simulink model "main"  (R2022a)
settings: Solver=FixedStepDiscrete  StartTime=0.0  StopTime=Inf  FixedStep=(50e-6)-(sim_en*4.995e-5)  RelTol=1e-3  EnableMultiTasking=on
model workspace (MAT data in the model file):
  Param : Simulink.Parameter (value not decoded)
  ac_ok : Simulink.Signal (value not decoded)
  ac_ok_120 : Simulink.Signal (value not decoded)
  bulk_voltage : Simulink.Signal (value not decoded)
  burstduty_integ_max : Simulink.Signal (value not decoded)
  burstduty_integ_min : Simulink.Signal (value not decoded)
  burstduty_ki : Simulink.Signal (value not decoded)
  burstduty_kp : Simulink.Signal (value not decoded)
  calib_ok : Simulink.Signal (value not decoded)
  can_addr1 : Simulink.Signal (value not decoded)
  can_addr2 : Simulink.Signal (value not decoded)
  can_addr3 : Simulink.Signal (value not decoded)
  can_addr4 : Simulink.Signal (value not decoded)
  can_data_rx : Simulink.Signal (value not decoded)
  can_data_tx : Simulink.Signal (value not decoded)
  can_timeout_120 : Simulink.Signal (value not decoded)
  chksum_scircv : Simulink.Signal (value not decoded)
  clllc_en_120 : Simulink.Signal (value not decoded)
  clllc_fault_120 : Simulink.Signal (value not decoded)
  clllc_ok_120 : Simulink.Signal (value not decoded)
  cmpss1h : Simulink.Signal (value not decoded)
  cmpss1l : Simulink.Signal (value not decoded)
  cmpss2h : Simulink.Signal (value not decoded)
  cmpss2l : Simulink.Signal (value not decoded)
  cmpss3h : Simulink.Signal (value not decoded)
  cmpss3l : Simulink.Signal (value not decoded)
  cmpss4h : Simulink.Signal (value not decoded)
  cmpss4l : Simulink.Signal (value not decoded)
  cmpss5h : Simulink.Signal (value not decoded)
  cmpss5l : Simulink.Signal (value not decoded)
  cmpss6h : Simulink.Signal (value not decoded)
  cmpss6l : Simulink.Signal (value not decoded)
  cmpss7h : Simulink.Signal (value not decoded)
  cmpss7l : Simulink.Signal (value not decoded)
  cmpss8h : Simulink.Signal (value not decoded)
  cmpss8l : Simulink.Signal (value not decoded)
  cnt_idle : Simulink.Signal (value not decoded)
  cnt_orps : Simulink.Signal (value not decoded)
  cnt_scircv : Simulink.Signal (value not decoded)
  cnt_scixmt : Simulink.Signal (value not decoded)
  cnt_scixmt_func : Simulink.Signal (value not decoded)
  cnt_temp_mux : Simulink.Signal (value not decoded)
  cnt_vdroop : Simulink.Signal (value not decoded)
  config_ok : Simulink.Signal (value not decoded)
  control_en : Simulink.Signal (value not decoded)
  cp_ready_120 : Simulink.Signal (value not decoded)
  d2d_en : Simulink.Signal (value not decoded)
  dchg_off : Simulink.Signal (value not decoded)
  debug_dacb : Simulink.Signal (value not decoded)
  debug_dacc : Simulink.Signal (value not decoded)
  debug_msg1 : Simulink.Signal (value not decoded)
  debug_msg2 : Simulink.Signal (value not decoded)
  debug_msg3 : Simulink.Signal (value not decoded)
  debug_msg4 : Simulink.Signal (value not decoded)
  debug_msg5 : Simulink.Signal (value not decoded)
  debug_msg6 : Simulink.Signal (value not decoded)
  dir_v2g : Simulink.Signal (value not decoded)
  eoss_llc1 : Simulink.Signal (value not decoded)
  eoss_llc2 : Simulink.Signal (value not decoded)
  eoss_orps : Simulink.Signal (value not decoded)
  fault_ocp : Simulink.Signal (value not decoded)
  fault_otp : Simulink.Signal (value not decoded)
  fault_ovp : Simulink.Signal (value not decoded)
  fut_en : Simulink.Signal (value not decoded)
  fwd_en_120 : Simulink.Signal (value not decoded)
  gain_llc1_sec_idc : Simulink.Signal (value not decoded)
  gain_llc1_temp_sr : Simulink.Signal (value not decoded)
  gain_llc2_sec_idc : Simulink.Signal (value not decoded)
  gain_vbat : Simulink.Signal (value not decoded)
  gain_vbulk : Simulink.Signal (value not decoded)
  gain_vout : Simulink.Signal (value not decoded)
  input_current_phasea : Simulink.Signal (value not decoded)
  input_current_phaseb : Simulink.Signal (value not decoded)
  input_current_phasec : Simulink.Signal (value not decoded)
  input_freq : Simulink.Signal (value not decoded)
  input_power : Simulink.Signal (value not decoded)
  input_voltage_phasea : Simulink.Signal (value not decoded)
  input_voltage_phaseb : Simulink.Signal (value not decoded)
  input_voltage_phasec : Simulink.Signal (value not decoded)
  ishare_arbiter : Simulink.Signal (value not decoded)
  ishare_thresh : Simulink.Signal (value not decoded)
  led_g : Simulink.Signal (value not decoded)
  led_r : Simulink.Signal (value not decoded)
  led_y : Simulink.Signal (value not decoded)
  llc1_burst_integ : Simulink.Signal (value not decoded)
  llc1_burstduty_buffer : Simulink.Signal (value not decoded)
  llc1_pfm_error : Simulink.Signal (value not decoded)
  llc1_pfm_integ : Simulink.Signal (value not decoded)
  llc1_pfm_prop : Simulink.Signal (value not decoded)
  llc1_pri_idc : Simulink.Signal (value not decoded)
  llc1_ps_buffer : Simulink.Signal (value not decoded)
  llc1_pspwm_error : Simulink.Signal (value not decoded)
  llc1_pspwm_integ : Simulink.Signal (value not decoded)
  llc1_pspwm_prop : Simulink.Signal (value not decoded)
  llc1_sec_idc : Simulink.Signal (value not decoded)
  llc1_temp_sr : Simulink.Signal (value not decoded)
  llc1_ts_tbctr_buffer : Simulink.Signal (value not decoded)
  llc2_burst_integ : Simulink.Signal (value not decoded)
  llc2_burstduty_buffer : Simulink.Signal (value not decoded)
  llc2_en : Simulink.Signal (value not decoded)
  llc2_en_buffer : Simulink.Signal (value not decoded)
  llc2_pfm_error : Simulink.Signal (value not decoded)
  llc2_pfm_integ : Simulink.Signal (value not decoded)
  llc2_pfm_prop : Simulink.Signal (value not decoded)
  llc2_pri_idc : Simulink.Signal (value not decoded)
  llc2_ps_buffer : Simulink.Signal (value not decoded)
  llc2_pspwm_error : Simulink.Signal (value not decoded)
  llc2_pspwm_integ : Simulink.Signal (value not decoded)
  llc2_pspwm_prop : Simulink.Signal (value not decoded)
  llc2_sec_idc : Simulink.Signal (value not decoded)
  llc2_temp_sr : Simulink.Signal (value not decoded)
  llc2_ts_tbctr_buffer : Simulink.Signal (value not decoded)
  loop_adcint : Simulink.Signal (value not decoded)
  loop_control : Simulink.Signal (value not decoded)
  loop_idle : Simulink.Signal (value not decoded)
  mid_bulk_voltage : Simulink.Signal (value not decoded)
  mode_120 : Simulink.Signal (value not decoded)
  mode_cc_cv : Simulink.Signal (value not decoded)
  myParam : mpt.Parameter (value not decoded)
  obc_ok_120 : Simulink.Signal (value not decoded)
  offset_llc1_sec_idc : Simulink.Signal (value not decoded)
  offset_llc1_temp_sr : Simulink.Signal (value not decoded)
  offset_llc2_sec_idc : Simulink.Signal (value not decoded)
  offset_vbat : Simulink.Signal (value not decoded)
  offset_vbulk : Simulink.Signal (value not decoded)
  offset_vout : Simulink.Signal (value not decoded)
  openloop_en : Simulink.Signal (value not decoded)
  openloop_fault_en : Simulink.Signal (value not decoded)
  ot_fault_120 : Simulink.Signal (value not decoded)
  pfc_en : Simulink.Signal (value not decoded)
  pfc_en_120 : Simulink.Signal (value not decoded)
  pfc_fw_revision : Simulink.Signal (value not decoded)
  pfc_fw_revision_bootloader : Simulink.Signal (value not decoded)
  pfc_fw_revision_debug : Simulink.Signal (value not decoded)
  pfc_ok : Simulink.Signal (value not decoded)
  pfc_ok_120 : Simulink.Signal (value not decoded)
  pfm_a0 : Simulink.Signal (value not decoded)
  pfm_a1 : Simulink.Signal (value not decoded)
  pfm_integ_max : Simulink.Signal (value not decoded)
  pfm_integ_min : Simulink.Signal (value not decoded)
  pfm_ki : Simulink.Signal (value not decoded)
  pfm_kp : Simulink.Signal (value not decoded)
  pri_fut_en : Simulink.Signal (value not decoded)
  pri_fut_en_buffer : Simulink.Signal (value not decoded)
  pri_halfbridge_en : Simulink.Signal (value not decoded)
  pri_halfbridge_en_buffer : Simulink.Signal (value not decoded)
  pspwm_integ_max : Simulink.Signal (value not decoded)
  pspwm_integ_min : Simulink.Signal (value not decoded)
  pspwm_ki : Simulink.Signal (value not decoded)
  pspwm_kp : Simulink.Signal (value not decoded)
  ref_idclink_max : Simulink.Signal (value not decoded)
  ref_iout : Simulink.Signal (value not decoded)
  ref_iout_calib : Simulink.Signal (value not decoded)
  ref_iout_llc1 : Simulink.Signal (value not decoded)
  ref_iout_llc1_calib : Simulink.Signal (value not decoded)
  ref_iout_llc2 : Simulink.Signal (value not decoded)
  ref_iout_llc2_calib : Simulink.Signal (value not decoded)
  ref_pout : Simulink.Signal (value not decoded)
  ref_ss_llc1 : Simulink.Signal (value not decoded)
  ref_ss_llc2 : Simulink.Signal (value not decoded)
  ref_ss_orps : Simulink.Signal (value not decoded)
  ref_vbat : Simulink.Signal (value not decoded)
  ref_vbat_calib : Simulink.Signal (value not decoded)
  ref_vbulk : Simulink.Signal (value not decoded)
  ref_vbulk_calib : Simulink.Signal (value not decoded)
  ref_vbulk_llc1_calib : Simulink.Signal (value not decoded)
  ref_vbulk_llc2_calib : Simulink.Signal (value not decoded)
  ref_vout : Simulink.Signal (value not decoded)
  ref_vout_calib : Simulink.Signal (value not decoded)
  relay_en : Simulink.Signal (value not decoded)
  reset_flag : Simulink.Signal (value not decoded)
  rev_en_120 : Simulink.Signal (value not decoded)
  runtime_control : Simulink.Signal (value not decoded)
  runtime_idle : Simulink.Signal (value not decoded)
  scircv_buffer : Simulink.Signal (value not decoded)
  scircv_buffer_tmp : Simulink.Signal (value not decoded)
  scircv_buffer_tmp_idx0 : Simulink.Signal (value not decoded)
  scircv_chksum : Simulink.Signal (value not decoded)
  scircv_chksum_ok : Simulink.Signal (value not decoded)
  scircv_parse_ok : Simulink.Signal (value not decoded)
  scixmt_buffer : Simulink.Signal (value not decoded)
  scixmt_chksum : Simulink.Signal (value not decoded)
  scixmt_func : Simulink.Signal (value not decoded)
  scixmt_word0_lsb : Simulink.Signal (value not decoded)
  scixmt_word0_msb : Simulink.Signal (value not decoded)
  scixmt_word1_lsb : Simulink.Signal (value not decoded)
  scixmt_word1_msb : Simulink.Signal (value not decoded)
  scixmt_word2_lsb : Simulink.Signal (value not decoded)
  scixmt_word2_msb : Simulink.Signal (value not decoded)
  scixmt_wr : Simulink.Signal (value not decoded)
  ss_step : Simulink.Signal (value not decoded)
  state_calib : Simulink.Signal (value not decoded)
  state_control : Simulink.Signal (value not decoded)
  state_hkeep : Simulink.Signal (value not decoded)
  status_cmpss : Simulink.Signal (value not decoded)
  status_control : Simulink.Signal (value not decoded)
  status_digin : Simulink.Signal (value not decoded)
  status_digout : Simulink.Signal (value not decoded)
  status_fault : Simulink.Signal (value not decoded)
  status_input : Simulink.Signal (value not decoded)
  status_pfc : Simulink.Signal (value not decoded)
  temp_inlet : Simulink.Signal (value not decoded)
  temp_llc1_fet_hs : Simulink.Signal (value not decoded)
  temp_llc2_fet_hs : Simulink.Signal (value not decoded)
  temp_mux : Simulink.Signal (value not decoded)
  temp_mux_s0 : Simulink.Signal (value not decoded)
  temp_mux_s1 : Simulink.Signal (value not decoded)
  temp_mux_s2 : Simulink.Signal (value not decoded)
  temp_outlet : Simulink.Signal (value not decoded)
  temp_pfc_fet_hsa : Simulink.Signal (value not decoded)
  temp_pfc_fet_hsb : Simulink.Signal (value not decoded)
  temp_pfc_fet_hsc : Simulink.Signal (value not decoded)
  temp_pfc_fet_lsa : Simulink.Signal (value not decoded)
  temp_pfc_fet_lsb : Simulink.Signal (value not decoded)
  temp_pfc_fet_lsc : Simulink.Signal (value not decoded)
  test_mode : Simulink.Signal (value not decoded)
  tfcv_cc : Simulink.Signal (value not decoded)
  tfcv_cc_llc2 : Simulink.Signal (value not decoded)
  tfcv_cv : Simulink.Signal (value not decoded)
  tfcv_sr_en : Simulink.Signal (value not decoded)
  tfv_assert_llc1_pri_idc : Simulink.Signal (value not decoded)
  tfv_assert_llc1_sec_idc : Simulink.Signal (value not decoded)
  tfv_assert_llc1_temp_sr : Simulink.Signal (value not decoded)
  tfv_assert_llc2_pri_idc : Simulink.Signal (value not decoded)
  tfv_assert_llc2_sec_idc : Simulink.Signal (value not decoded)
  tfv_assert_llc2_temp_sr : Simulink.Signal (value not decoded)
  tfv_assert_temp_outlet : Simulink.Signal (value not decoded)
  tfv_assert_vaux_uv : Simulink.Signal (value not decoded)
  tfv_assert_vbat : Simulink.Signal (value not decoded)
  tfv_assert_vbulk : Simulink.Signal (value not decoded)
  tfv_assert_vout : Simulink.Signal (value not decoded)
  tfv_cnt_tz : Simulink.Signal (value not decoded)
  tfv_deassert_llc1_pri_idc : Simulink.Signal (value not decoded)
  tfv_deassert_llc1_sec_idc : Simulink.Signal (value not decoded)
  tfv_deassert_llc1_temp_sr : Simulink.Signal (value not decoded)
  tfv_deassert_llc2_pri_idc : Simulink.Signal (value not decoded)
  tfv_deassert_llc2_sec_idc : Simulink.Signal (value not decoded)
  tfv_deassert_llc2_temp_sr : Simulink.Signal (value not decoded)
  tfv_deassert_temp_outlet : Simulink.Signal (value not decoded)
  tfv_deassert_vaux_uv : Simulink.Signal (value not decoded)
  tfv_deassert_vbat : Simulink.Signal (value not decoded)
  tfv_deassert_vbulk : Simulink.Signal (value not decoded)
  tfv_deassert_vout : Simulink.Signal (value not decoded)
  tfv_llc1_pri_idc : Simulink.Signal (value not decoded)
  tfv_llc1_sec_idc : Simulink.Signal (value not decoded)
  tfv_llc1_temp_sr : Simulink.Signal (value not decoded)
  tfv_llc2_pri_idc : Simulink.Signal (value not decoded)
  tfv_llc2_sec_idc : Simulink.Signal (value not decoded)
  tfv_llc2_temp_sr : Simulink.Signal (value not decoded)
  tfv_temp_outlet : Simulink.Signal (value not decoded)
  tfv_vaux_uv : Simulink.Signal (value not decoded)
  tfv_vbat : Simulink.Signal (value not decoded)
  tfv_vbulk : Simulink.Signal (value not decoded)
  tfv_vout : Simulink.Signal (value not decoded)
  timer_1ms : Simulink.Signal (value not decoded)
  tz : Simulink.Signal (value not decoded)
  valve_en : Simulink.Signal (value not decoded)
  vaux : Simulink.Signal (value not decoded)
  vbat : Simulink.Signal (value not decoded)
  vbulk : Simulink.Signal (value not decoded)
  vout : Simulink.Signal (value not decoded)
undefined symbols (not defined in the file or in its folder): CAN_O_INT, CANA_BASE, Down, GPTRIP1SEL, GPTRIP2SEL, TZ1, TZ2, Up
libraries: hdlsllib x159, simulink x100, c2837xDlib x24, c2807xlib x16, c280xlib x13, c2802xlib x12, canmsglib x8, idelinklib_common x2, c2000lib x1, c281xlib x1
(part 7 of 15)

== system main/Task_Manager/idle/idle_task/uartx/parse ==
  function : TriggerPort  TriggerType=function-call  VariantControl=Variant
  System Outputs3 : Subsystem  mask(System Outputs){ShowInLibBrowser=0}
      mask prompts: ShowInLibBrowser "Simulink:masks:CustCodeMaskParam1_MP"
      settings: CopyFcn=cccopyfcn(gcb)  OpenFcn=ccopenfcn('System Outputs Function')
      mask Help: eval('feval(''rtwprivate'',''rtwhelpview'',''rtw_sys_outputs_block'')');
      mask Display: disp('System\nOutputs');

== system main/Task_Manager/idle/idle_task/uartx/uart_xmt ==
  function : TriggerPort  TriggerType=function-call  VariantControl=Variant

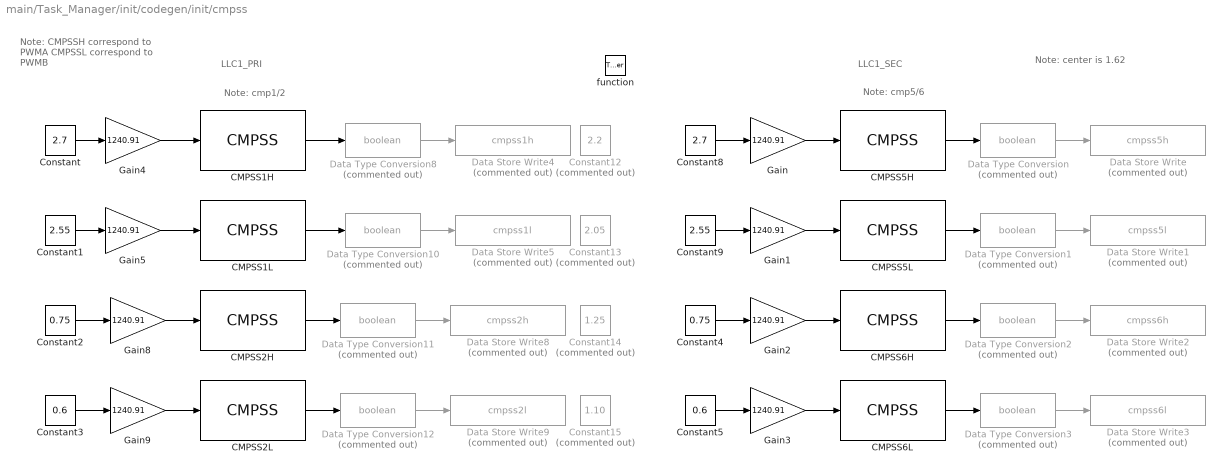
== system main/Task_Manager/init/codegen/init/cmpss ==
  note: Note:
      | center is 1.62
  note: Note:
      | CMPSSH correspond to PWMA
      | CMPSSL correspond to PWMB
  note: LLC1_PRI
  note: LLC1_SEC
  note: Note: cmp1/2
  note: Note: cmp5/6
  function : TriggerPort  TriggerType=function-call  VariantControl=Variant
  CMPSS1H : c2837xDlib/CMPSS  Module=CMPSS1_COMPH  NegativeInput=Internal DAC  DacValueSourceSel=DAC module  DacValueVia=Input port  DACHValue=2234  DACLValue=0  RampMaxRefVal=0  RampDecVal=0  RampDelayVal=0  EnableLatchOut=off  EnableLatchClear=off  SampleTime=-1
      settings: SourceProductBaseCode=TIC2000
  CMPSS1L : c2837xDlib/CMPSS  Module=CMPSS1_COMPL  NegativeInput=Internal DAC  DacValueSourceSel=DAC module  DacValueVia=Input port  DACHValue=2234  DACLValue=0  RampMaxRefVal=0  RampDecVal=0  RampDelayVal=0  EnableLatchOut=off  EnableLatchClear=off  SampleTime=-1
      settings: SourceProductBaseCode=TIC2000
  CMPSS2H : c2837xDlib/CMPSS  Module=CMPSS2_COMPH  NegativeInput=Internal DAC  DacValueSourceSel=DAC module  DacValueVia=Input port  DACHValue=2234  DACLValue=0  RampMaxRefVal=0  RampDecVal=0  RampDelayVal=0  EnableLatchOut=off  EnableLatchClear=off  SampleTime=-1
      settings: SourceProductBaseCode=TIC2000
  CMPSS2L : c2837xDlib/CMPSS  Module=CMPSS2_COMPL  NegativeInput=Internal DAC  DacValueSourceSel=DAC module  DacValueVia=Input port  DACHValue=2234  DACLValue=0  RampMaxRefVal=0  RampDecVal=0  RampDelayVal=0  EnableLatchOut=off  EnableLatchClear=off  SampleTime=-1
      settings: SourceProductBaseCode=TIC2000
  CMPSS5H : c2837xDlib/CMPSS  Module=CMPSS5_COMPH  NegativeInput=Internal DAC  DacValueSourceSel=DAC module  DacValueVia=Input port  DACHValue=2234  DACLValue=0  RampMaxRefVal=0  RampDecVal=0  RampDelayVal=0  EnableLatchOut=off  EnableLatchClear=off  SampleTime=-1
      settings: SourceProductBaseCode=TIC2000
  CMPSS5L : c2837xDlib/CMPSS  Module=CMPSS5_COMPL  NegativeInput=Internal DAC  DacValueSourceSel=DAC module  DacValueVia=Input port  DACHValue=2234  DACLValue=0  RampMaxRefVal=0  RampDecVal=0  RampDelayVal=0  EnableLatchOut=off  EnableLatchClear=off  SampleTime=-1
      settings: SourceProductBaseCode=TIC2000
  CMPSS6H : c2837xDlib/CMPSS  Module=CMPSS6_COMPH  NegativeInput=Internal DAC  DacValueSourceSel=DAC module  DacValueVia=Input port  DACHValue=2234  DACLValue=0  RampMaxRefVal=0  RampDecVal=0  RampDelayVal=0  EnableLatchOut=off  EnableLatchClear=off  SampleTime=-1
      settings: SourceProductBaseCode=TIC2000
  CMPSS6L : c2837xDlib/CMPSS  Module=CMPSS6_COMPL  NegativeInput=Internal DAC  DacValueSourceSel=DAC module  DacValueVia=Input port  DACHValue=2234  DACLValue=0  RampMaxRefVal=0  RampDecVal=0  RampDelayVal=0  EnableLatchOut=off  EnableLatchClear=off  SampleTime=-1
      settings: SourceProductBaseCode=TIC2000
  Constant : Constant  Value=2.7
  Constant1 : Constant  Value=2.55
  Constant12 : Constant  Commented=on  Value=2.2
  Constant13 : Constant  Commented=on  Value=2.05
  Constant14 : Constant  Commented=on  Value=1.25
  Constant15 : Constant  Commented=on  Value=1.10
  Constant2 : Constant  Value=0.75
  Constant3 : Constant  Value=0.6
  Constant4 : Constant  Value=0.75
  Constant5 : Constant  Value=0.6
  Constant8 : Constant  Value=2.7
  Constant9 : Constant  Value=2.55
  Data Store Write : DataStoreWrite  Commented=on  DataStoreName=cmpss5h  IndexOptions=Index vector (dialog)  Indices=1  OutputSizes=1
  Data Store Write1 : DataStoreWrite  Commented=on  DataStoreName=cmpss5l  IndexOptions=Index vector (dialog)  Indices=1  OutputSizes=1
  Data Store Write2 : DataStoreWrite  Commented=on  DataStoreName=cmpss6h  IndexOptions=Index vector (dialog)  Indices=1  OutputSizes=1
  Data Store Write3 : DataStoreWrite  Commented=on  DataStoreName=cmpss6l  IndexOptions=Index vector (dialog)  Indices=1  OutputSizes=1
  Data Store Write4 : DataStoreWrite  Commented=on  DataStoreName=cmpss1h  IndexOptions=Index vector (dialog)  Indices=1  OutputSizes=1
  Data Store Write5 : DataStoreWrite  Commented=on  DataStoreName=cmpss1l  IndexOptions=Index vector (dialog)  Indices=1  OutputSizes=1
  Data Store Write8 : DataStoreWrite  Commented=on  DataStoreName=cmpss2h  IndexOptions=Index vector (dialog)  Indices=1  OutputSizes=1
  Data Store Write9 : DataStoreWrite  Commented=on  DataStoreName=cmpss2l  IndexOptions=Index vector (dialog)  Indices=1  OutputSizes=1
  Data Type Conversion{,1..3,8,10..12} (8 alike) : DataTypeConversion  Commented=on  OutDataTypeStr=boolean  SaturateOnIntegerOverflow=off  RndMeth=Floor
  Gain{,1..5,8..9} (8 alike) : Gain  Gain=1240.91
  wires:
  Constant/1 -> Gain4/1
  Constant1/1 -> Gain5/1
  Gain/1 -> CMPSS5H/1
  Gain1/1 -> CMPSS5L/1
  Gain2/1 -> CMPSS6H/1
  Gain3/1 -> CMPSS6L/1
  CMPSS5H/1 -> Data Type Conversion/1
  CMPSS5L/1 -> Data Type Conversion1/1
  CMPSS6H/1 -> Data Type Conversion2/1
  CMPSS6L/1 -> Data Type Conversion3/1
  CMPSS1H/1 -> Data Type Conversion8/1
  CMPSS1L/1 -> Data Type Conversion10/1
  Gain4/1 -> CMPSS1H/1
  Gain5/1 -> CMPSS1L/1
  CMPSS2L/1 -> Data Type Conversion12/1
  CMPSS2H/1 -> Data Type Conversion11/1
  Gain9/1 -> CMPSS2L/1
  Gain8/1 -> CMPSS2H/1
  Constant3/1 -> Gain9/1
  Constant2/1 -> Gain8/1
  Data Type Conversion/1 -> Data Store Write/1
  Data Type Conversion1/1 -> Data Store Write1/1
  Data Type Conversion3/1 -> Data Store Write3/1
  Data Type Conversion2/1 -> Data Store Write2/1
  Data Type Conversion8/1 -> Data Store Write4/1
  Data Type Conversion10/1 -> Data Store Write5/1
  Data Type Conversion11/1 -> Data Store Write8/1
  Data Type Conversion12/1 -> Data Store Write9/1
  Constant4/1 -> Gain2/1
  Constant5/1 -> Gain3/1
  Constant9/1 -> Gain1/1
  Constant8/1 -> Gain/1

== system main/Task_Manager/init/codegen/init/orps&relay ==
  note: Note:
      | Period: 100kHz
      |
      | Timer Period: 1000
      |
      | ePWM9 GPIO16
  function : TriggerPort  TriggerType=function-call  VariantControl=Variant
  ORPS : c2802xlib/ePWM  PwmType=C2000_Type4  useModule=ePWM9  ePWMxLINKTBPRD=Not Linked  periodUnits=Clock cycles  timerSource=Specify via dialog  timerPeriod_clk=1000  timerPeriod_sec=0.0001  tbshadow=Counter equals to zero  countingMode=Up-Down  phaseActiveEnable=Disable  phaseDirection=Count down after sync  phaseActive=0  synchronizationEnable=off  dcaevt1Sync=off  dcbevt1Sync=off  synchronizationOption=Pass through (EPWMxSYNCI or SWFSYNC)  perSynchronizationOption=Counter equals to period (CTR=PRD)  clockPrescale=1  HSclockPrescale=1  enswap=off  ePWMxAStatus=on  ePWMxAactionLogic1=Set  ePWMxAactionLogic2=Do nothing  ePWMxAactionLogic3=Do nothing  ePWMxAactionLogic4=Do nothing  ePWMxAactionLogic5=Clear  ePWMxAactionLogic6=Do nothing  ePWMxACSFenable=off  ePWMxACSFvalue=Forcing disable  ePWMxASFreload=Zero  ePWMxBStatus=on  ePWMxBactionLogic1=Do nothing  ePWMxBactionLogic2=Set  ePWMxBactionLogic3=Do nothing  ePWMxBactionLogic4=Clear  ePWMxBactionLogic5=Do nothing  ePWMxBactionLogic6=Do nothing  ePWMxBCSFenable=off  ePWMxBCSFvalue=Forcing disable  ePWMxBSFreload=Zero  ePWNxBOutWay=off  ePWMxLINKCMPA=Not Linked  CMPAUnits=Clock cycles  CMPASource=Specify via dialog  CMPAValue_per=50  CMPAValue_clk=5  enCMPAshadow=Counter equals to zero (CTR=Zero)  ePWMxLINKCMPB=Not Linked  CMPBUnits=Clock cycles  CMPBSource=Specify via dialog  CMPBValue_per=50  CMPBValue_clk=995  enCMPBshadow=Counter equals to zero (CTR=Zero)  ePWMxLINKCMPC=Not Linked  CMPCUnits=Clock cycles  CMPCSource=Specify via dialog  CMPCValue_per=50  CMPCValue_clk=0  enCMPCshadow=Counter equals to zero (CTR=Zero)  ePWMxLINKCMPD=Not Linked  CMPDUnits=Clock cycles  CMPDSource=Specify via dialog  CMPDValue_per=50  CMPDValue_clk=0  enCMPDshadow=Counter equals to zero (CTR=Zero)  enableDBePWMxA=off  enableDBePWMxB=off  enhalfcycle=off  DBpolarity=Active high complementary (AHC)  DBedgeDelay=Positive  DBSource_ePWMxA=ePWMxA  DBSource_ePWMxB=ePWMxA  DBPeriodUnits=Clock cycles  DBperiodSource=Input port  REDperiod=36  FEDperiod=36  REDperiod_sec=0  FEDperiod_sec=0  LoadModeDBRED=Immediate without using shadow  LoadModeDBFED=Immediate without using shadow  adcstartModuleA=off  adcrequestEventA=First event  adcstartEventA=Digital Compare Module A Event 1 start of conversion (DCAEVT1.soc)  adcstartEventA_type2=Counter is incrementing and equals to the compare B register (CTRU=CMPB)  adcstartModuleB=off  adcrequestEventB=First event  adcstartEventB=Counter equals to zero (CTR=Zero)  adcstartEventB_type2=Counter is incrementing and equals to the compare B register (CTRU=CMPB)  intEn=off  intPrd=First event  intSel=Counter equals to zero (CTR=Zero)  intSel_type2=Counter equals to zero (CTR=Zero)  hrpe=off  enHRPWM=off  HRPWM_LoadMode=Counter equals to period (CTR=PRD)  HRPWM_CTLMode=Duty or Period control mode  HRPWM_EDGMode=Both edge  hrpeb=off  enHRPWMB=off  HRPWM_LoadModeB=Counter equals to zero (CTR=ZERO)  HRPWM_CTLModeB=Duty or Period control mode  HRPWM_EDGModeB=Both edge  enHRDBRED=off  enHRDBFED=off  enSFO=on  enautoconv=on  chopperEnable=off  chopperFrequency=1  chopperFirstwidth=1  chopperDuty=12.5%  tripZonesource=Specify via dialog  tzselOSHT1=off  tzselOSHT2=off  tzselOSHT3=off  tzselOSHDCAEV1=off  tzselOSHDCBEV1=off  tzselCBC1=off  tzselCBC2=off  tzselCBC3=off  tzselCBCDCAEV2=off  tzselCBCDCBEV2=off  tzselOSHT4=off  tzselOSHT5=off  tzselOSHT6=off  tzselCBC4=off  tzselCBC5=off  tzselCBC6=off  enTzOstIntr=off  enTzCbcIntr=off  enTzDCAEVT1Intr=off  enTzDCAEVT2Intr=off  enTzDCBEVT1Intr=off  enTzDCBEVT2Intr=off  ePWMxAforced=No action  ePWMxBforced=No action  DCAEVT1forced=High  DCBEVT1forced=Low  DCAEVT2forced=Low  DCBEVT2forced=High  dcah=Trip Zone 1 input (TZ1)  dcal=Trip Zone 2 input (TZ2)  dcbh=Trip Zone 1 input (TZ1)  dcbl=Trip Zone 2 input (TZ2)  dcah_type2=GPTRIP4SEL  dcal_type2=GPTRIP4SEL  dcbh_type2=GPTRIP5SEL  dcbl_type2=GPTRIP5SEL  gendcaevt1=Event disabled  gendcaevt2=Event disabled  gendcbevt1=Event disabled  gendcbevt2=Event disabled  dcaevt1src=DCAEVT1 with sync  dcaevt2src=DCAEVT2 with sync  dcbevt1src=DCBEVT1 with sync  dcbevt2src=DCBEVT2 with sync  pulsesel=Counter equals to zero (CTR=Zero)  blankinv=off  blankoffset=0  blankwidth=0  evsrcsel=Filtered version of DCAEVT1 (DCAEVT1FILT)  encape=off

== system main/Task_Manager/init/codegen/init/outputxbar ==
  note: //Code:
      | GPIO_setPinConfig(GPIO_24_OUTPUTXBAR1);
      | GPIO_setDirectionMode(24, GPIO_DIR_MODE_OUT);
      | GPIO_setPadConfig(24, GPIO_PIN_TYPE_STD);
      | XBAR_setOutputMuxConfig(XBAR_OUTPUT1, XBAR_OUT_MUX00_CMPSS1_CTRIPOUTH);
      | XBAR_enableOutputMux(XBAR_OUTPUT1, XBAR_MUX00);
      |
      | GPIO_setPinConfig(GPIO_25_OUTPUTXBAR2);
      | GPIO_setDirectionMode(25, GPIO_DIR_MODE_OUT);
      | GPIO_setPadConfig(25, GPIO_PIN_TYPE_STD);
      | XBAR_setOutputMuxConfig(XBAR_OUTPUT2, XBAR_OUT_MUX01_CMPSS1_CTRIPOUTL);
      | XBAR_enableOutputMux(XBAR_OUTPUT2, XBAR_MUX01);
      |
      | GPIO_setPinConfig(GPIO_26_OUTPUTXBAR3);
      | GPIO_setDirectionMode(26, GPIO_DIR_MODE_OUT);
      | GPIO_setPadConfig(26, GPIO_PIN_TYPE_STD);
      | XBAR_setOutputMuxConfig(XBAR_OUTPUT3, XBAR_OUT_MUX04_CMPSS3_CTRIPOUTH);
      | XBAR_enableOutputMux(XBAR_OUTPUT3, XBAR_MUX04);
      |
      | GPIO_setPinConfig(GPIO_27_OUTPUTXBAR4);
      | GPIO_setDirectionMode(27, GPIO_DIR_MODE_OUT);
      | GPIO_setPadConfig(27, GPIO_PIN_TYPE_STD);
      | XBAR_setOutputMuxConfig(XBAR_OUTPUT4, XBAR_OUT_MUX05_CMPSS3_CTRIPOUTL);
      | XBAR_enableOutputMux(XBAR_OUTPUT4, XBAR_MUX05);
  note: GPIO_setPinConfig(GPIO_24_OUTPUTXBAR1);
      | GPIO_setDirectionMode(24, GPIO_DIR_MODE_OUT);
      | GPIO_setPadConfig(24, GPIO_PIN_TYPE_STD);
      | XBAR_setOutputMuxConfig(XBAR_OUTPUT1, XBAR_OUT_MUX11_CMPSS6_CTRIPOUTL);
      | XBAR_enableOutputMux(XBAR_OUTPUT1, XBAR_MUX11);
      |
      | GPIO_setPinConfig(GPIO_25_OUTPUTXBAR2);
      | GPIO_setDirectionMode(25, GPIO_DIR_MODE_OUT);
      | GPIO_setPadConfig(25, GPIO_PIN_TYPE_STD);
      | XBAR_setOutputMuxConfig(XBAR_OUTPUT2, XBAR_OUT_MUX10_CMPSS6_CTRIPOUTH);
      | XBAR_enableOutputMux(XBAR_OUTPUT2, XBAR_MUX10);
  note: GPIO_setPinConfig(GPIO_24_OUTPUTXBAR1);
      | GPIO_setDirectionMode(24, GPIO_DIR_MODE_OUT);
      | GPIO_setPadConfig(24, GPIO_PIN_TYPE_STD);
      | XBAR_setOutputMuxConfig(XBAR_OUTPUT1, XBAR_CLB_MUX08_CMPSS5_CTRIPH);
      | XBAR_enableOutputMux(XBAR_OUTPUT1, XBAR_MUX08);
  note: GPIO_setPinConfig(GPIO_24_OUTPUTXBAR1);
      | GPIO_setDirectionMode(24, GPIO_DIR_MODE_OUT);
      | GPIO_setPadConfig(24, GPIO_PIN_TYPE_STD);
      | XBAR_setOutputMuxConfig(XBAR_OUTPUT1, XBAR_CLB_MUX00_CMPSS1_CTRIPH);
      | XBAR_enableOutputMux(XBAR_OUTPUT1, XBAR_MUX00);
  note: GPIO_setPinConfig(GPIO_25_OUTPUTXBAR2);
      | GPIO_setDirectionMode(25, GPIO_DIR_MODE_OUT);
      | GPIO_setPadConfig(25, GPIO_PIN_TYPE_STD);
      | XBAR_setOutputMuxConfig(XBAR_OUTPUT2, XBAR_CLB_MUX00_CMPSS1_CTRIPH);
      | XBAR_enableOutputMux(XBAR_OUTPUT2, XBAR_MUX00);
  note: GPIO_setPinConfig(GPIO_25_OUTPUTXBAR2);
      | GPIO_setDirectionMode(25, GPIO_DIR_MODE_OUT);
      | GPIO_setPadConfig(25, GPIO_PIN_TYPE_STD);
      | XBAR_setOutputMuxConfig(XBAR_OUTPUT2, XBAR_CLB_MUX08_CMPSS5_CTRIPH);
      | XBAR_enableOutputMux(XBAR_OUTPUT2, XBAR_MUX08);
  function : TriggerPort  TriggerType=function-call  VariantControl=Variant
  System Initialize1 : Subsystem  Commented=on  mask(System Initialize){ShowInLibBrowser=0}
      mask prompts: ShowInLibBrowser "Simulink:masks:CustCodeMaskParam1_MP"
      settings: CopyFcn=cccopyfcn(gcb)  OpenFcn=ccopenfcn('System Initialize Function')
      mask Help: eval('feval(''rtwprivate'',''rtwhelpview'',''rtw_sys_initialize_block'')');
      mask Display: disp('System\nInitialize');
  System Initialize2 : Subsystem  Commented=on  mask(System Initialize){ShowInLibBrowser=0}
      mask prompts: ShowInLibBrowser "Simulink:masks:CustCodeMaskParam1_MP"
      settings: CopyFcn=cccopyfcn(gcb)  OpenFcn=ccopenfcn('System Initialize Function')
      mask Help: eval('feval(''rtwprivate'',''rtwhelpview'',''rtw_sys_initialize_block'')');
      mask Display: disp('System\nInitialize');
  System Initialize3 : Subsystem  Commented=on  mask(System Initialize){ShowInLibBrowser=0}
      mask prompts: ShowInLibBrowser "Simulink:masks:CustCodeMaskParam1_MP"
      settings: CopyFcn=cccopyfcn(gcb)  OpenFcn=ccopenfcn('System Initialize Function')
      mask Help: eval('feval(''rtwprivate'',''rtwhelpview'',''rtw_sys_initialize_block'')');
      mask Display: disp('System\nInitialize');
  System Initialize4 : Subsystem  Commented=on  mask(System Initialize){ShowInLibBrowser=0}
      mask prompts: ShowInLibBrowser "Simulink:masks:CustCodeMaskParam1_MP"
      settings: CopyFcn=cccopyfcn(gcb)  OpenFcn=ccopenfcn('System Initialize Function')
      mask Help: eval('feval(''rtwprivate'',''rtwhelpview'',''rtw_sys_initialize_block'')');
      mask Display: disp('System\nInitialize');
  System Initialize5 : Subsystem  Commented=on  mask(System Initialize){ShowInLibBrowser=0}
      mask prompts: ShowInLibBrowser "Simulink:masks:CustCodeMaskParam1_MP"
      settings: CopyFcn=cccopyfcn(gcb)  OpenFcn=ccopenfcn('System Initialize Function')
      mask Help: eval('feval(''rtwprivate'',''rtwhelpview'',''rtw_sys_initialize_block'')');
      mask Display: disp('System\nInitialize');
  System Initialize6 : Subsystem  mask(System Initialize){ShowInLibBrowser=0}
      mask prompts: ShowInLibBrowser "Simulink:masks:CustCodeMaskParam1_MP"
      settings: CopyFcn=cccopyfcn(gcb)  OpenFcn=ccopenfcn('System Initialize Function')
      mask Help: eval('feval(''rtwprivate'',''rtwhelpview'',''rtw_sys_initialize_block'')');
      mask Display: disp('System\nInitialize');

== system main/Task_Manager/init/codegen/init/pwmsync ==
  note: EALLOW;
      | XBAR_setInputPin(XBAR_INPUT5, 4); //EXTSYNC1 from PWM3A
      | XBAR_setInputPin(XBAR_INPUT6, 10); //EXTSYNC2 from PWM6A
      | EDIS;
  note: Note:
      | grouping is:
      |
      | 1/2            7/8
      |
      | 4/5            10/11
  note: EALLOW;
      | SyncSocRegs.SYNCSELECT.bit.EPWM4SYNCIN = 0b110; //Sync to PWM4 group to EXTSYNC2
      | EDIS;
  note: EALLOW;
      | XBAR_setInputPin(XBAR_INPUT5, 4); //EXTSYNC1 from PWM3A
      | SyncSocRegs.SYNCSELECT.bit.EPWM7SYNCIN = 0b101; //Sync PWM7 group to EXTSYNC1
      | EDIS;
  note: Note:
      | grouping is:
      | Use external sync
      |
      | 1/2            7/8
      |
      | epwm9 for orps
  function : TriggerPort  TriggerType=function-call  VariantControl=Variant
  System Initialize : Subsystem  Commented=on  mask(System Initialize){ShowInLibBrowser=0}
      mask prompts: ShowInLibBrowser "Simulink:masks:CustCodeMaskParam1_MP"
      settings: CopyFcn=cccopyfcn(gcb)  OpenFcn=ccopenfcn('System Initialize Function')
      mask Help: eval('feval(''rtwprivate'',''rtwhelpview'',''rtw_sys_initialize_block'')');
      mask Display: disp('System\nInitialize');
  System Initialize1 : Subsystem  Commented=on  mask(System Initialize){ShowInLibBrowser=0}
      mask prompts: ShowInLibBrowser "Simulink:masks:CustCodeMaskParam1_MP"
      settings: CopyFcn=cccopyfcn(gcb)  OpenFcn=ccopenfcn('System Initialize Function')
      mask Help: eval('feval(''rtwprivate'',''rtwhelpview'',''rtw_sys_initialize_block'')');
      mask Display: disp('System\nInitialize');
  System Initialize2 : Subsystem  mask(System Initialize){ShowInLibBrowser=0}
      mask prompts: ShowInLibBrowser "Simulink:masks:CustCodeMaskParam1_MP"
      settings: CopyFcn=cccopyfcn(gcb)  OpenFcn=ccopenfcn('System Initialize Function')
      mask Help: eval('feval(''rtwprivate'',''rtwhelpview'',''rtw_sys_initialize_block'')');
      mask Display: disp('System\nInitialize');

== system main/Task_Manager/init/codegen/init/tztl_clb ==
  note: Note:
      | Initial configuration is for
      | G2V full-bridge
  function : TriggerPort  TriggerType=function-call  VariantControl=Variant
  Function-Call Generator1 : simulink/Ports & Subsystems/Function-Call Generator  sample_time=-1  numberOfIterations=1  DisallowWideOutput=off
  Function-Call Split3 : FunctionCallSplit  NumOutputPorts=2
  clb : Subsystem  TreatAsAtomicUnit=on
      settings: RTWSystemCode=Inline
  tzctl : Subsystem  TreatAsAtomicUnit=on
      settings: RTWSystemCode=Inline
  wires:
  Function-Call Split3/2 -> clb/Trigger
  Function-Call Generator1/1 -> Function-Call Split3/1
  Function-Call Split3/1 -> tzctl/Trigger

== system main/interrupt_adcd/burst_control/burst/enPulse/Forward/System Outputs1 ==

== system main/interrupt_adcd/burst_control/burst/enPulse/Reverse/System Outputs1 ==

== system main/interrupt_canrx/canrx_variant_subsystem/codegen/can_rcv/Switch Case Action Subsystem ==
  Action Port : ActionPort  ActionPortLabel=case [ 10 ]:
  Constant : Constant  OutDataTypeStr=boolean
  Data Store Write : DataStoreWrite  DataStoreName=u8CanDataRx10  IndexOptions=Index vector (dialog)  Indices=1  OutputSizes=1
  Data Store Write1 : DataStoreWrite  DataStoreName=b05_MB10Received  IndexOptions=Index vector (dialog)  Indices=1  OutputSizes=1
  Terminator : Terminator
  eCAN Receive : c280xlib/eCAN Receive  chipFamily=C280x  useModule=eCAN_A  mailboxNo=9  messageID=hex2dec('00000100')  messageType=Standard (11-bit identifier)  enableAcceptanceFiltering=off  messageIDMask=0  sampleTime=-1  dataType=uint8  outputAction=Output last received values  initValue=0  outputMessageID=off  outputMessageLength=off  outputMessageTimeStamp=off  postInterrupt=on  interruptLine=0
      settings: SourceProductBaseCode=TIC2000
  wires:
  eCAN Receive/2 -> Data Store Write/1
  eCAN Receive/1 -> Terminator/1
  Constant/1 -> Data Store Write1/1

== system main/interrupt_canrx/canrx_variant_subsystem/codegen/can_rcv/Switch Case Action Subsystem1 ==
  Action Port : ActionPort  ActionPortLabel=case [ 11 ]:
  Constant2 : Constant  OutDataTypeStr=boolean
  Data Store Write1 : DataStoreWrite  DataStoreName=b06_MB11Received  IndexOptions=Index vector (dialog)  Indices=1  OutputSizes=1
  Data Store Write3 : DataStoreWrite  DataStoreName=u8CanDataRx11  IndexOptions=Index vector (dialog)  Indices=1  OutputSizes=1
  Terminator1 : Terminator
  eCAN Receive1 : c280xlib/eCAN Receive  chipFamily=C280x  useModule=eCAN_A  mailboxNo=10  messageID=hex2dec('00000102')  messageType=Standard (11-bit identifier)  enableAcceptanceFiltering=off  messageIDMask=0  sampleTime=-1  dataType=uint8  outputAction=Output last received values  initValue=0  outputMessageID=off  outputMessageLength=off  outputMessageTimeStamp=off  postInterrupt=on  interruptLine=0
      settings: SourceProductBaseCode=TIC2000
  wires:
  eCAN Receive1/1 -> Terminator1/1
  eCAN Receive1/2 -> Data Store Write3/1
  Constant2/1 -> Data Store Write1/1

== system main/interrupt_canrx/canrx_variant_subsystem/codegen/can_rcv/Switch Case Action Subsystem2 ==
  Action Port : ActionPort  ActionPortLabel=case [ 12 ]:
  Constant2 : Constant  OutDataTypeStr=boolean
  Data Store Write1 : DataStoreWrite  DataStoreName=u8CanDataRx12  IndexOptions=Index vector (dialog)  Indices=1  OutputSizes=1
  Data Store Write2 : DataStoreWrite  DataStoreName=b07_MB12Received  IndexOptions=Index vector (dialog)  Indices=1  OutputSizes=1
  Terminator2 : Terminator
  eCAN Receive2 : c280xlib/eCAN Receive  chipFamily=C280x  useModule=eCAN_A  mailboxNo=11  messageID=hex2dec('0000010A')  messageType=Standard (11-bit identifier)  enableAcceptanceFiltering=off  messageIDMask=0  sampleTime=-1  dataType=uint8  outputAction=Output last received values  initValue=0  outputMessageID=off  outputMessageLength=off  outputMessageTimeStamp=off  postInterrupt=on  interruptLine=0
      settings: SourceProductBaseCode=TIC2000
  wires:
  eCAN Receive2/1 -> Terminator2/1
  eCAN Receive2/2 -> Data Store Write1/1
  Constant2/1 -> Data Store Write2/1

== system main/Control_State_Machine/Control_Loop/control/configSr/configXbarEpwmtrip/codegen/g2v_prifullbridge ==
  Action Port : ActionPort
  Function-Call Generator1 : simulink/Ports & Subsystems/Function-Call Generator  sample_time=-1  numberOfIterations=1  DisallowWideOutput=off
  Function-Call Split3 : FunctionCallSplit  NumOutputPorts=2
  clb : Subsystem  TreatAsAtomicUnit=on
      settings: RTWSystemCode=Inline
  tzctl : Subsystem  TreatAsAtomicUnit=on
      settings: RTWSystemCode=Inline
  wires:
  Function-Call Split3/1 -> tzctl/Trigger
  Function-Call Generator1/1 -> Function-Call Split3/1
  Function-Call Split3/2 -> clb/Trigger

== system main/Control_State_Machine/Control_Loop/control/configSr/configXbarEpwmtrip/codegen/v2g_prifullbridge ==
  Action Port : ActionPort
  Function-Call Generator2 : simulink/Ports & Subsystems/Function-Call Generator  sample_time=-1  numberOfIterations=1  DisallowWideOutput=off
  Function-Call Split1 : FunctionCallSplit  NumOutputPorts=2
  clb : Subsystem  TreatAsAtomicUnit=on
      settings: RTWSystemCode=Inline
  tzctl : Subsystem  TreatAsAtomicUnit=on
      settings: RTWSystemCode=Inline
  wires:
  Function-Call Generator2/1 -> Function-Call Split1/1
  Function-Call Split1/1 -> tzctl/Trigger
  Function-Call Split1/2 -> clb/Trigger

== system main/Control_State_Machine/Control_Loop/control/configSr/configXbarEpwmtrip/sim/g2v_prifullbridge ==
  Action Port : ActionPort
  Constant{,1..3} (4 alike) : Constant  Value=0  OutDataTypeStr=uint16
  Constant{4,9..11} (4 alike) : Constant  OutDataTypeStr=uint16
  Data Store Write1 : DataStoreWrite  DataStoreName=xbar_epwmtrip_llc1_pri_qb_en  IndexOptions=Index vector (dialog)  Indices=1  OutputSizes=1
  Data Store Write10 : DataStoreWrite  DataStoreName=xbar_epwmtrip_llc1_sec_qd_en  IndexOptions=Index vector (dialog)  Indices=1  OutputSizes=1
  Data Store Write2 : DataStoreWrite  DataStoreName=xbar_epwmtrip_llc1_pri_qc_en  IndexOptions=Index vector (dialog)  Indices=1  OutputSizes=1
  Data Store Write3 : DataStoreWrite  DataStoreName=xbar_epwmtrip_llc1_pri_qd_en  IndexOptions=Index vector (dialog)  Indices=1  OutputSizes=1
  Data Store Write4 : DataStoreWrite  DataStoreName=xbar_epwmtrip_llc1_sec_qa_en  IndexOptions=Index vector (dialog)  Indices=1  OutputSizes=1
  Data Store Write6 : DataStoreWrite  DataStoreName=xbar_epwmtrip_llc1_pri_qa_en  IndexOptions=Index vector (dialog)  Indices=1  OutputSizes=1
  Data Store Write8 : DataStoreWrite  DataStoreName=xbar_epwmtrip_llc1_sec_qb_en  IndexOptions=Index vector (dialog)  Indices=1  OutputSizes=1
  Data Store Write9 : DataStoreWrite  DataStoreName=xbar_epwmtrip_llc1_sec_qc_en  IndexOptions=Index vector (dialog)  Indices=1  OutputSizes=1
  wires:
  Constant3/1 -> Data Store Write3/1
  Constant2/1 -> Data Store Write2/1
  Constant1/1 -> Data Store Write1/1
  Constant/1 -> Data Store Write6/1
  Constant4/1 -> Data Store Write4/1
  Constant9/1 -> Data Store Write8/1
  Constant10/1 -> Data Store Write9/1
  Constant11/1 -> Data Store Write10/1

== system main/Control_State_Machine/Control_Loop/control/configSr/configXbarEpwmtrip/sim/v2g_prifullbridge ==
  Action Port : ActionPort
  Constant{,1..3} (4 alike) : Constant  Value=0  OutDataTypeStr=uint16
  Constant{4,9..11} (4 alike) : Constant  OutDataTypeStr=uint16
  Data Store Write1 : DataStoreWrite  DataStoreName=xbar_epwmtrip_llc1_pri_qb_en  IndexOptions=Index vector (dialog)  Indices=1  OutputSizes=1
  Data Store Write10 : DataStoreWrite  DataStoreName=xbar_epwmtrip_llc1_sec_qd_en  IndexOptions=Index vector (dialog)  Indices=1  OutputSizes=1
  Data Store Write2 : DataStoreWrite  DataStoreName=xbar_epwmtrip_llc1_pri_qc_en  IndexOptions=Index vector (dialog)  Indices=1  OutputSizes=1
  Data Store Write3 : DataStoreWrite  DataStoreName=xbar_epwmtrip_llc1_pri_qd_en  IndexOptions=Index vector (dialog)  Indices=1  OutputSizes=1
  Data Store Write4 : DataStoreWrite  DataStoreName=xbar_epwmtrip_llc1_sec_qa_en  IndexOptions=Index vector (dialog)  Indices=1  OutputSizes=1
  Data Store Write6 : DataStoreWrite  DataStoreName=xbar_epwmtrip_llc1_pri_qa_en  IndexOptions=Index vector (dialog)  Indices=1  OutputSizes=1
  Data Store Write8 : DataStoreWrite  DataStoreName=xbar_epwmtrip_llc1_sec_qb_en  IndexOptions=Index vector (dialog)  Indices=1  OutputSizes=1
  Data Store Write9 : DataStoreWrite  DataStoreName=xbar_epwmtrip_llc1_sec_qc_en  IndexOptions=Index vector (dialog)  Indices=1  OutputSizes=1
  wires:
  Constant4/1 -> Data Store Write6/1
  Constant11/1 -> Data Store Write3/1
  Constant10/1 -> Data Store Write2/1
  Constant9/1 -> Data Store Write1/1
  Constant1/1 -> Data Store Write8/1
  Constant2/1 -> Data Store Write9/1
  Constant3/1 -> Data Store Write10/1
  Constant/1 -> Data Store Write4/1

== system main/Task_Manager/Tmr_1mS/codegen/Task_1mS/GPIO_Handler/Update_ACOK ==
  Dig_Input : Inport  OutDataTypeStr=boolean
  Constant : Constant  Value=10  OutDataTypeStr=uint16
  Constant1 : Constant  Value=10  OutDataTypeStr=uint16
  Constant2 : Constant  OutDataTypeStr=boolean
  Validate_DI : MATLABSystem  System=Validate_DI  SimulateUsing=Code generation
      mask Type: Validate_DI
      mask Display:
      | disp('Validate_DI');
      | port_label('input',1,'din');
      | port_label('input',2,'assert_logic');
      | port_label('input',3,'assert_dly');
      | port_label('input',4,'deassert_dly');
      | port_label('output',1,'status');
  Dig_Input_State : Outport  OutDataTypeStr=boolean
  wires:
  Validate_DI/1 -> Dig_Input_State/1
  Constant2/1 -> Validate_DI/2
  Constant1/1 -> Validate_DI/4
  Constant/1 -> Validate_DI/3
  Dig_Input/1 -> Validate_DI/1

== system main/Task_Manager/Tmr_1mS/codegen/Task_1mS/GPIO_Handler/Update_CLLLCEN ==
  Dig_Input : Inport  OutDataTypeStr=boolean
  Constant : Constant  Value=10  OutDataTypeStr=uint16
  Constant1 : Constant  Value=10  OutDataTypeStr=uint16
  Constant2 : Constant  OutDataTypeStr=boolean
  Validate_DI : MATLABSystem  System=Validate_DI  SimulateUsing=Code generation
      mask Type: Validate_DI
      mask Display:
      | disp('Validate_DI');
      | port_label('input',1,'din');
      | port_label('input',2,'assert_logic');
      | port_label('input',3,'assert_dly');
      | port_label('input',4,'deassert_dly');
      | port_label('output',1,'status');
  Dig_Input_State : Outport  OutDataTypeStr=boolean
  wires:
  Validate_DI/1 -> Dig_Input_State/1
  Constant2/1 -> Validate_DI/2
  Constant1/1 -> Validate_DI/4
  Constant/1 -> Validate_DI/3
  Dig_Input/1 -> Validate_DI/1

== system main/Task_Manager/Tmr_1mS/codegen/Task_1mS/GPIO_Handler/Update_CPReady ==
  Dig_Input : Inport  OutDataTypeStr=boolean
  Constant : Constant  Value=10  OutDataTypeStr=uint16
  Constant1 : Constant  Value=10  OutDataTypeStr=uint16
  Constant2 : Constant  OutDataTypeStr=boolean
  Validate_DI : MATLABSystem  System=Validate_DI  SimulateUsing=Code generation
      mask Type: Validate_DI
      mask Display:
      | disp('Validate_DI');
      | port_label('input',1,'din');
      | port_label('input',2,'assert_logic');
      | port_label('input',3,'assert_dly');
      | port_label('input',4,'deassert_dly');
      | port_label('output',1,'status');
  Dig_Input_State : Outport  OutDataTypeStr=boolean
  wires:
  Validate_DI/1 -> Dig_Input_State/1
  Dig_Input/1 -> Validate_DI/1
  Constant/1 -> Validate_DI/3
  Constant1/1 -> Validate_DI/4
  Constant2/1 -> Validate_DI/2

== system main/Task_Manager/Tmr_1mS/codegen/Task_1mS/GPIO_Handler/Update_PFCOK ==
  Dig_Input : Inport  OutDataTypeStr=boolean
  Constant : Constant  Value=10  OutDataTypeStr=uint16
  Constant1 : Constant  Value=10  OutDataTypeStr=uint16
  Constant2 : Constant  OutDataTypeStr=boolean
  Validate_DI : MATLABSystem  System=Validate_DI  SimulateUsing=Code generation
      mask Type: Validate_DI
      mask Display:
      | disp('Validate_DI');
      | port_label('input',1,'din');
      | port_label('input',2,'assert_logic');
      | port_label('input',3,'assert_dly');
      | port_label('input',4,'deassert_dly');
      | port_label('output',1,'status');
  Dig_Input_State : Outport  OutDataTypeStr=boolean
  wires:
  Validate_DI/1 -> Dig_Input_State/1
  Dig_Input/1 -> Validate_DI/1
  Constant/1 -> Validate_DI/3
  Constant1/1 -> Validate_DI/4
  Constant2/1 -> Validate_DI/2

== system main/Task_Manager/Tmr_1s/codegen/Task_1S/addressing_temp_mux/cnt_temp_mux0 ==
  Action Port : ActionPort  ActionPortLabel=if(u1 == 0)
  Constant : Constant  Value=0  OutDataTypeStr=boolean
  Constant1 : Constant  Value=0  OutDataTypeStr=boolean
  Constant2 : Constant  Value=0  OutDataTypeStr=boolean
  Data Store Write : DataStoreWrite  DataStoreName=temp_mux_s0  IndexOptions=Index vector (dialog)  Indices=1  OutputSizes=1
  Data Store Write1 : DataStoreWrite  DataStoreName=temp_mux_s1  IndexOptions=Index vector (dialog)  Indices=1  OutputSizes=1
  Data Store Write2 : DataStoreWrite  DataStoreName=temp_mux_s2  IndexOptions=Index vector (dialog)  Indices=1  OutputSizes=1
  wires:
  Constant1/1 -> Data Store Write1/1
  Constant2/1 -> Data Store Write2/1
  Constant/1 -> Data Store Write/1

== system main/Task_Manager/Tmr_1s/codegen/Task_1S/addressing_temp_mux/cnt_temp_mux1 ==
  Action Port : ActionPort  ActionPortLabel=elseif(u1 == 1)
  Constant : Constant  Value=0  OutDataTypeStr=boolean
  Constant1 : Constant  OutDataTypeStr=boolean
  Constant2 : Constant  Value=0  OutDataTypeStr=boolean
  Data Store Write : DataStoreWrite  DataStoreName=temp_mux_s0  IndexOptions=Index vector (dialog)  Indices=1  OutputSizes=1
  Data Store Write1 : DataStoreWrite  DataStoreName=temp_mux_s1  IndexOptions=Index vector (dialog)  Indices=1  OutputSizes=1
  Data Store Write2 : DataStoreWrite  DataStoreName=temp_mux_s2  IndexOptions=Index vector (dialog)  Indices=1  OutputSizes=1
  wires:
  Constant/1 -> Data Store Write/1
  Constant2/1 -> Data Store Write2/1
  Constant1/1 -> Data Store Write1/1

== system main/Task_Manager/Tmr_1s/codegen/Task_1S/addressing_temp_mux/cnt_temp_mux2 ==
  Action Port : ActionPort  ActionPortLabel=elseif( u1 == 2)
  Constant : Constant  Value=0  OutDataTypeStr=boolean
  Constant1 : Constant  OutDataTypeStr=boolean
  Constant2 : Constant  OutDataTypeStr=boolean
  Data Store Write : DataStoreWrite  DataStoreName=temp_mux_s0  IndexOptions=Index vector (dialog)  Indices=1  OutputSizes=1
  Data Store Write1 : DataStoreWrite  DataStoreName=temp_mux_s1  IndexOptions=Index vector (dialog)  Indices=1  OutputSizes=1
  Data Store Write2 : DataStoreWrite  DataStoreName=temp_mux_s2  IndexOptions=Index vector (dialog)  Indices=1  OutputSizes=1
  wires:
  Constant/1 -> Data Store Write/1
  Constant2/1 -> Data Store Write2/1
  Constant1/1 -> Data Store Write1/1

== system main/Task_Manager/Tmr_1s/codegen/Task_1S/cnt_temp_mux/cnt_temp_mux ==
  Action Port : ActionPort  ActionPortLabel=if(u1 < 3)
  Add : Sum
  Constant : Constant  OutDataTypeStr=uint16
  Data Store Read1 : DataStoreRead  DataStoreName=cnt_temp_mux  IndexOptions=Index vector (dialog)  Indices=1  OutputSizes=1
  Data Store Write : DataStoreWrite  DataStoreName=cnt_temp_mux  IndexOptions=Index vector (dialog)  Indices=1  OutputSizes=1
  wires:
  Data Store Read1/1 -> Add/1
  Add/1 -> Data Store Write/1
  Constant/1 -> Add/2

== system main/Task_Manager/Tmr_1s/codegen/Task_1S/cnt_temp_mux/cnt_temp_mux_sat ==
  Action Port : ActionPort  ActionPortLabel=else
  Constant : Constant  Value=0  OutDataTypeStr=uint16
  Data Store Write : DataStoreWrite  DataStoreName=cnt_temp_mux  IndexOptions=Index vector (dialog)  Indices=1  OutputSizes=1
  wires:
  Constant/1 -> Data Store Write/1
